simulink library "heatGenerationForCellResolvedModel"  (R2025a)
settings: Solver=VariableStepAuto  StartTime=0.0  StopTime=10.0  RelTol=1e-3
settings Model: Creator=mbhattu  LastModifiedBy=mbhattu

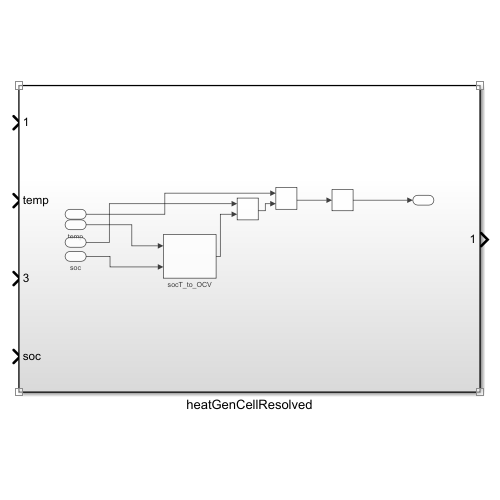
[thumbnail: Simulink's stored preview of the top-level diagram]
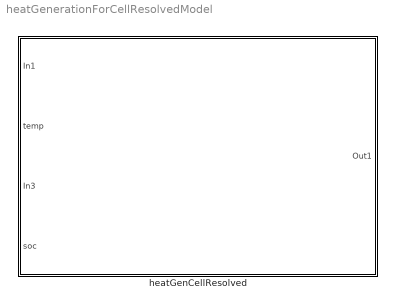
== system heatGenerationForCellResolvedModel ==
  heatGenCellResolved : Subsystem

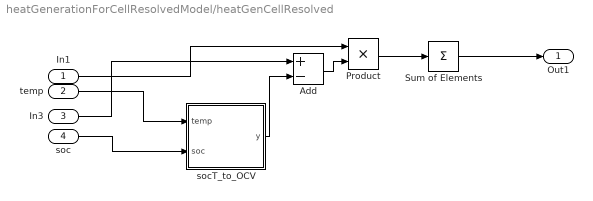
== system heatGenerationForCellResolvedModel/heatGenCellResolved ==
  In1 : Inport
  temp : Inport  Port=2
  In3 : Inport  Port=3
  soc : Inport  Port=4
  Add : Sum  Inputs=+-
  Product : Product
  Sum of Elements : Sum  Inputs=+
  socT_to_OCV : MATLAB Function  TreatAsAtomicUnit=on
  Out1 : Outport
  wires:
  Add/1 -> Product/2
  socT_to_OCV/1(y) -> Add/2
  Sum of Elements/1 -> Out1/1
  soc/1 -> socT_to_OCV/2(soc)
  In1/1 -> Product/1
  Product/1 -> Sum of Elements/1
  In3/1 -> Add/1
  temp/1 -> socT_to_OCV/1(temp)

== matlab function heatGenerationForCellResolvedModel/heatGenCellResolved/socT_to_OCV ==
  data: temp input; y output; soc input
function y = socT_to_OCV(temp, soc)

socBreaks = 0:0.05:1;
tempBreaks = [283.15; 298.15; 328.15];
ocvTable = [2.500,  2.500,  2.500;
    3.420,	3.386,	3.338;
    3.464,	3.428,	3.409;
    3.520,	3.481,	3.460;
    3.568,	3.535,	3.519;
    3.597,	3.577,	3.564;
    3.623,	3.606,	3.612;
    3.651,	3.642,	3.639;
    3.681,	3.671,	3.669;
    3.721,	3.707,	3.703;
    3.777,	3.753,	3.746;
    3.835,	3.817,	3.824;
    3.879,	3.864,	3.868;
    3.915,	3.903,	3.905;
    3.946,	3.944,	3.936;
    3.990,	3.988,	3.977;
    4.044,	4.041,	4.046;
    4.080,	4.077,	4.078;
    4.097,	4.092,	4.091;
    4.126,	4.116,	4.114;
    4.177,	4.132,	4.114];

F = griddedInterpolant({socBreaks, tempBreaks}, ocvTable, 'linear', 'nearest');

% Pairwise query (12×1 inputs give 12×1 outputs)
y = F(soc, temp);
end
